simulink model "MultiPortSwitch"  (R2020a)
settings: Solver=VariableStepAuto  StartTime=0.0  StopTime=10.0  RelTol=1e-3
settings Model: Creator=ashok  LastModifiedBy=ashok
settings DataIOCC: ExternalInput=[t,Input1,Input2,Input3,Input4,Input5]  LoadExternalInput=on

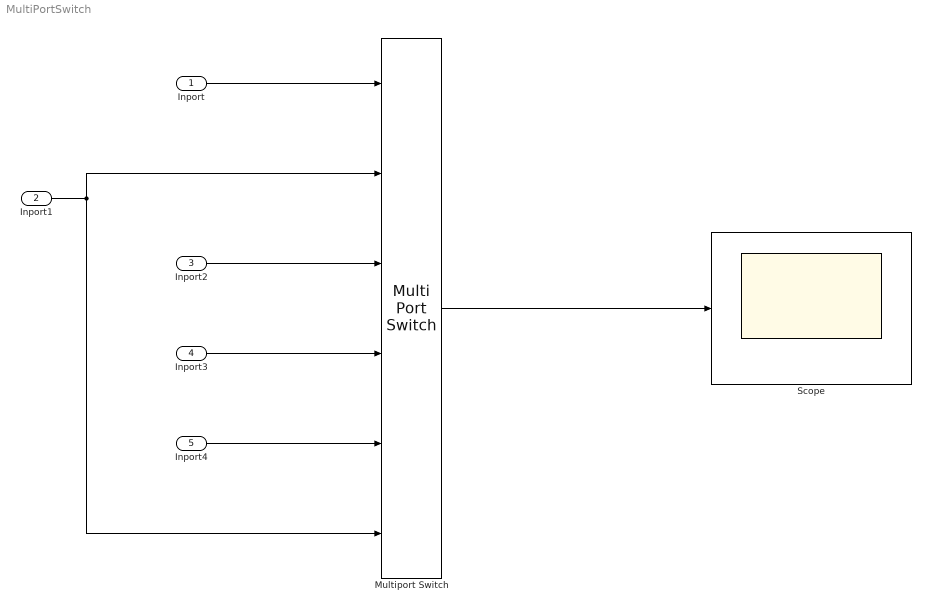
== system MultiPortSwitch ==
  Inport : Inport
  Inport1 : Inport  Port=2
  Inport2 : Inport  Port=3
  Inport3 : Inport  Port=4
  Inport4 : Inport  Port=5
  Multiport Switch : MultiPortSwitch  Inputs=4  DataPortForDefault=Additional data port  DiagnosticForDefault=Warning
  Scope : Scope
  wires:
  Multiport Switch/1 -> Scope/1
  Inport/1 -> Multiport Switch/1
  Inport1/1 -> Multiport Switch/2, Multiport Switch/6
  Inport2/1 -> Multiport Switch/3
  Inport3/1 -> Multiport Switch/4
  Inport4/1 -> Multiport Switch/5
